simulink model "sampleModel246"  (R2021b)
settings: Solver=VariableStepAuto  StartTime=0.0  StopTime=10.0  RelTol=1e-3
libraries: simulink x5
settings Model: Creator=user  LastModifiedBy=user

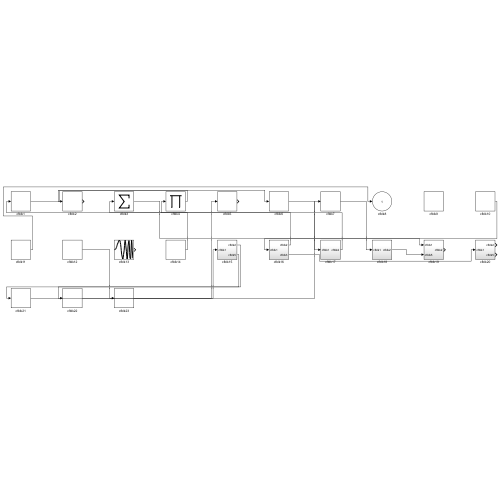
[thumbnail: Simulink's stored preview of the top-level diagram]
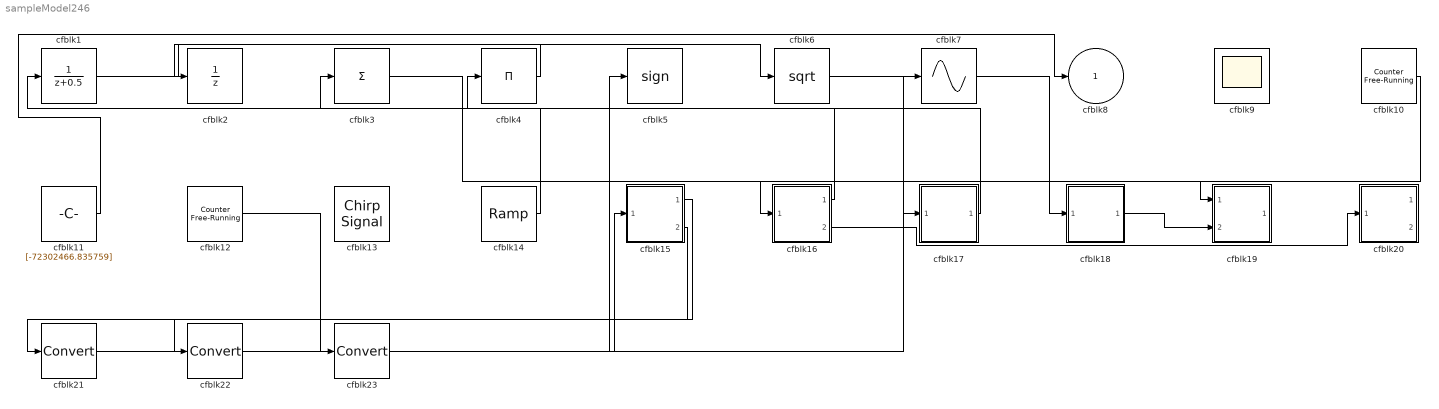
== system sampleModel246 ==
  cfblk1 : DiscreteTransferFcn  SampleTime=1
  cfblk10 : simulink/Sources/Counter Free-Running  NumBits=[19.000000]  tsamp=-1
  cfblk11 : Constant  Value=[-72302466.835759]  SampleTime=1
  cfblk12 : simulink/Sources/Counter Free-Running  NumBits=[21.000000]  tsamp=-1
  cfblk13 : simulink/Sources/Chirp Signal  f1=[258834182.589123]  T=[-821499069.196127]  f2=[-285450871.165295]
  cfblk14 : simulink/Sources/Ramp  slope=[-2001.948137]  start=[9.316688]  InitialOutput=[-735706.291074]
  cfblk15 : Subsystem
  cfblk16 : Subsystem
  cfblk17 : Subsystem
  cfblk18 : Subsystem
  cfblk19 : Subsystem
  cfblk2 : UnitDelay  HasFrameUpgradeWarning=on
  cfblk20 : Subsystem
  cfblk21 : DataTypeConversion
  cfblk22 : DataTypeConversion
  cfblk23 : DataTypeConversion
  cfblk3 : Sum  Inputs=+
  cfblk4 : Product  Inputs=*
  cfblk5 : Signum
  cfblk6 : Sqrt  SaturateOnIntegerOverflow=on
  cfblk7 : Sin  TimeSource=Use external signal  SampleTime=0
  cfblk9 : Scope
      settings: Floating=on
  cfblk8 : Outport
  wires:
  cfblk10/1 -> cfblk16/1(cfblk1)
  cfblk14/1 -> cfblk1/1
  cfblk1/1 -> cfblk6/1
  cfblk16/1(cfblk2) -> cfblk4/1
  cfblk6/1 -> cfblk17/1(cfblk1)
  cfblk17/1(cfblk2) -> cfblk3/1
  cfblk11/1 -> cfblk8/1
  cfblk16/2(cfblk3) -> cfblk20/1(cfblk1)
  cfblk4/1 -> cfblk2/1
  cfblk7/1 -> cfblk18/1(cfblk1)
  cfblk3/1 -> cfblk19/1(cfblk1)
  cfblk18/1(cfblk2) -> cfblk19/2(cfblk5)
  cfblk15/1(cfblk2) -> cfblk21/1
  cfblk21/1 -> cfblk7/1
  cfblk15/2(cfblk5) -> cfblk22/1
  cfblk22/1 -> cfblk5/1
  cfblk12/1 -> cfblk23/1
  cfblk23/1 -> cfblk15/1(cfblk1)

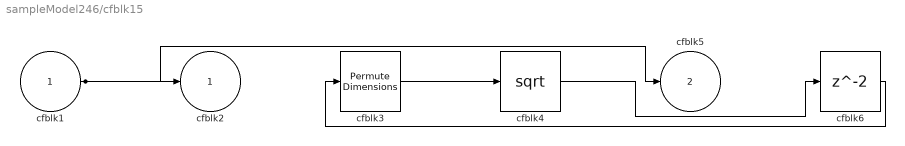
== system sampleModel246/cfblk15 ==
  cfblk1 : Inport
  cfblk3 : PermuteDimensions
  cfblk4 : Sqrt  SaturateOnIntegerOverflow=on
  cfblk6 : Delay  SampleTime=1
  cfblk2 : Outport
  cfblk5 : Outport  Port=2
  wires:
  cfblk1/1 -> cfblk2/1, cfblk5/1
  cfblk3/1 -> cfblk4/1
  cfblk4/1 -> cfblk6/1
  cfblk6/1 -> cfblk3/1

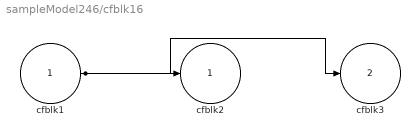
== system sampleModel246/cfblk16 ==
  cfblk1 : Inport
  cfblk2 : Outport
  cfblk3 : Outport  Port=2
  wires:
  cfblk1/1 -> cfblk3/1, cfblk2/1

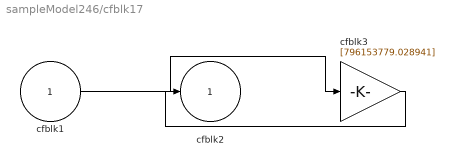
== system sampleModel246/cfblk17 ==
  cfblk1 : Inport
  cfblk3 : Gain  Gain=[796153779.028941]
  cfblk2 : Outport
  wires:
  cfblk1/1 -> cfblk3/1
  cfblk3/1 -> cfblk2/1

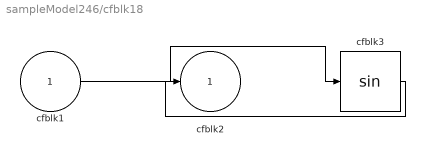
== system sampleModel246/cfblk18 ==
  cfblk1 : Inport
  cfblk3 : Trigonometry
  cfblk2 : Outport
  wires:
  cfblk1/1 -> cfblk3/1
  cfblk3/1 -> cfblk2/1

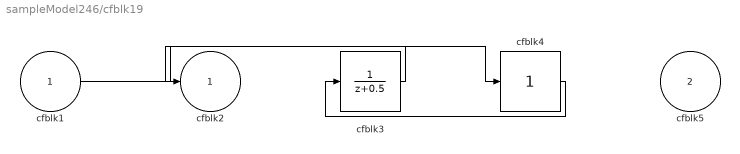
== system sampleModel246/cfblk19 ==
  cfblk1 : Inport
  cfblk5 : Inport  Port=2
  cfblk3 : DiscreteTransferFcn  SampleTime=1
  cfblk4 : simulink/Math Operations/Slider Gain  gain=1  low=0  high=2
  cfblk2 : Outport
  wires:
  cfblk1/1 -> cfblk4/1
  cfblk4/1 -> cfblk3/1
  cfblk3/1 -> cfblk2/1

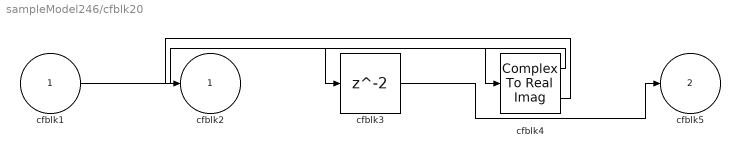
== system sampleModel246/cfblk20 ==
  cfblk1 : Inport
  cfblk3 : Delay  SampleTime=1
  cfblk4 : ComplexToRealImag
  cfblk2 : Outport
  cfblk5 : Outport  Port=2
  wires:
  cfblk1/1 -> cfblk4/1
  cfblk3/1 -> cfblk5/1
  cfblk4/1 -> cfblk3/1
  cfblk4/2 -> cfblk2/1
